simulink model "MCAN_EXTERNAL_READ_WRITE_AM261"  (R2024b)
settings: Solver=FixedStepAuto  StartTime=0.0  StopTime=10.0  RelTol=1e-3
libraries: peripheral_library_blocks_am261x x4, HWI_lib x1
settings Model: Creator=a0499511  LastModifiedBy=a0499511
settings OptimizationCC: DefaultParameterBehavior=Inlined  EnhancedBackFolding=on  PassReuseOutputArgsAs=Individual arguments  ZeroExternalMemoryAtStartup=off  ZeroInternalMemoryAtStartup=off  MaxStackSize=64  OptimizeBlockOrder=speed  DifferentSizesBufferReuse=on  OptimizationCustomize=off  EfficientTunableParamExpr=on
settings DebuggingCC: ParameterTunabilityLossMsg=error
settings HardwareCC: ProdBitPerPointer=32  ProdBitPerSizeT=32  ProdBitPerPtrDiffT=32  ProdLargestAtomicInteger=Long  ProdLargestAtomicFloat=Double  ProdWordSize=32  ProdHWDeviceType=ARM Compatible->ARM Cortex
settings SFSimCC: MATLABDynamicMemAlloc=off
settings RTWCC: Description=Embedded Coder  SystemTargetFile=ert.tlc  HardwareBoard=AM261X LP  TemplateMakefile=ert_default_tmf  Toolchain=TI ARM Clang Compiler AM261x | gmake
settings CodeAppCC: ForceParamTrailComments=on  IgnoreCustomStorageClasses=off  OperatorAnnotations=on  SimulinkDataObjDesc=on  SFDataObjDesc=on  InsertBlockDesc=on
settings ERTTargetCC: SupportVariableSizeSignals=on  ExtModeTransport=3  ExtModeStaticAlloc=on  ExtModeMexFile=ext_xcp  ExtModeIntrfLevel=Level2 - Open  ERTCustomFileTemplate=AM263x_codertarget_file_process.tlc

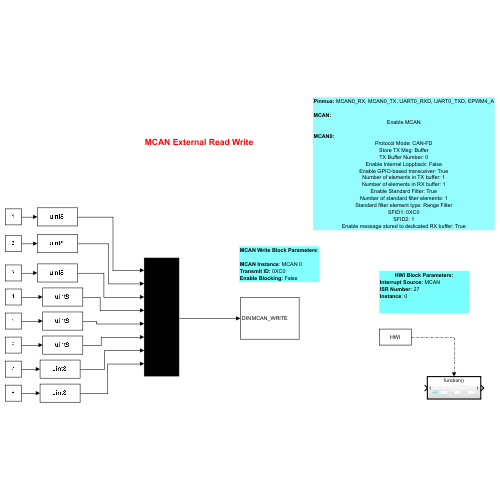
[thumbnail: Simulink's stored preview of the top-level diagram]
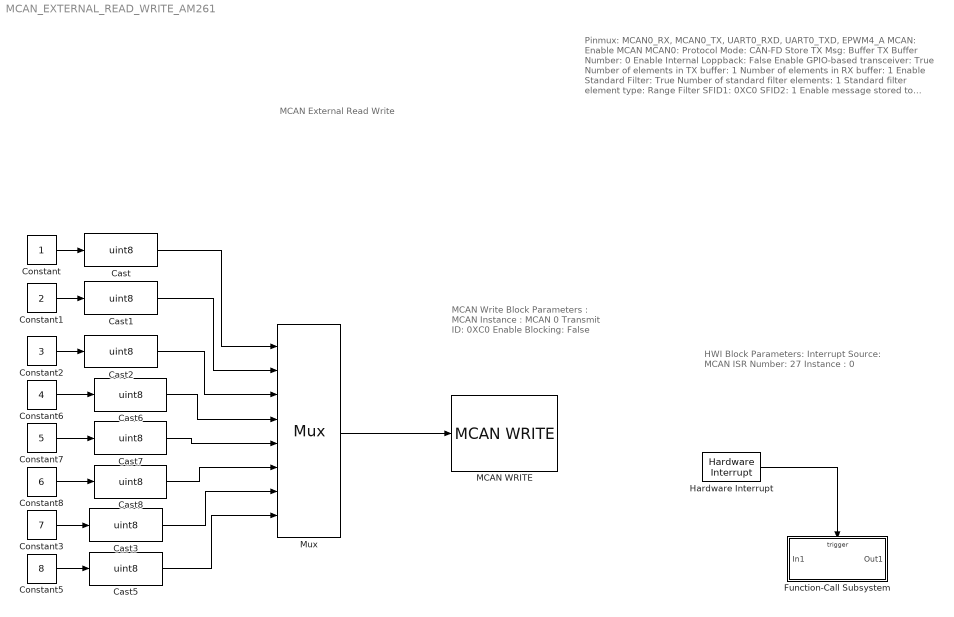
== system MCAN_EXTERNAL_READ_WRITE_AM261 ==
  note: MCAN External Read Write
  note: MCAN Write Block Parameters :
      |
      | MCAN Instance : MCAN 0
      | Transmit ID: 0XC0
      | Enable Blocking: False
  note: Pinmux: MCAN0_RX, MCAN0_TX, UART0_RXD, UART0_TXD, EPWM4_A
      |
      | MCAN:
      | Enable MCAN
      |
      | MCAN0:
      | Protocol Mode: CAN-FD
      | Store TX Msg: Buffer
      | TX Buffer Number: 0
      | Enable Internal Loppback: False
      | Enable GPIO-based transceiver: True
      | Number of elements in TX buffer: 1
      | Number of elements in RX buffer: 1
      | Enable Standard Filter: True
      | Number of standard filter elements: 1
      | Standard filter element type: Range Filter
      | SFID1: 0XC0
      | SFID2: 1
      | Enable message stored to dedicated RX buffer: True
  note: HWI Block Parameters:
      | Interrupt Source: MCAN
      | ISR Number: 27
      | Instance : 0
  Cast{,1..3,5..8} (8 alike) : DataTypeConversion  OutDataTypeStr=uint8  SaturateOnIntegerOverflow=off  RndMeth=Floor
  Constant : Constant
  Constant1 : Constant  Value=2
  Constant2 : Constant  Value=3
  Constant3 : Constant  Value=7
  Constant5 : Constant  Value=8
  Constant6 : Constant  Value=4
  Constant7 : Constant  Value=5
  Constant8 : Constant  Value=6
  Function-Call Subsystem : Subsystem  TreatAsAtomicUnit=on
  Hardware Interrupt : HWI_lib/Hardware Interrupt  INTERRUPT_TYPE=MCAN  ISR_NUMBER=68  INSTANCE_NUMBER=0  SHOW_INPUTPORT=off
      settings: SourceProductName=Embedded Coder Support Package for AM263x - HWI Block
  MCAN WRITE : peripheral_library_blocks_am261x/MCAN WRITE  MCAN_Instance=MCAN0  TX_MsgID=0xC0  Blocking_mode_tx=off
  Mux : Mux  Inputs=8
  wires:
  Cast3/1 -> Mux/7
  Constant8/1 -> Cast8/1
  Cast/1 -> Mux/1
  Constant6/1 -> Cast6/1
  Cast7/1 -> Mux/5
  Mux/1 -> MCAN WRITE/1
  Constant/1 -> Cast/1
  Hardware Interrupt/1 -> Function-Call Subsystem/Trigger
  Constant3/1 -> Cast3/1
  Cast1/1 -> Mux/2
  Constant5/1 -> Cast5/1
  Cast2/1 -> Mux/3
  Constant2/1 -> Cast2/1
  Cast5/1 -> Mux/8
  Cast8/1 -> Mux/6
  Constant1/1 -> Cast1/1
  Constant7/1 -> Cast7/1
  Cast6/1 -> Mux/4

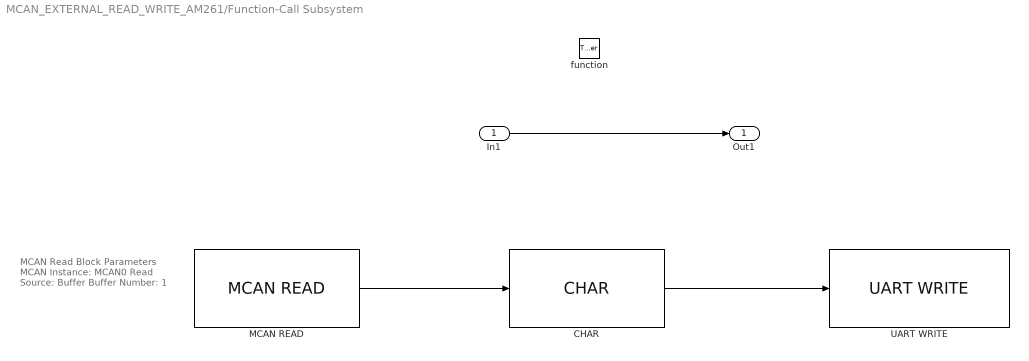
== system MCAN_EXTERNAL_READ_WRITE_AM261/Function-Call Subsystem ==
  note: MCAN Read Block Parameters
      |
      | MCAN Instance: MCAN0
      | Read Source: Buffer
      | Buffer Number: 1
  In1 : Inport
  function : TriggerPort  TriggerType=function-call  VariantControl=(inherit)
  CHAR : peripheral_library_blocks_am261x/CHAR
  MCAN READ : peripheral_library_blocks_am261x/MCAN READ  MCAN_Instance=MCAN0  Enable_blockingrx=off  Read_src=Buffer  Buffer_num=1  Enable_OutputPort=on  SampleTime=-1
  UART WRITE : peripheral_library_blocks_am261x/UART WRITE  UARTPort=UART0
  Out1 : Outport
  wires:
  In1/1 -> Out1/1
  MCAN READ/1 -> CHAR/1
  CHAR/1 -> UART WRITE/1
